simulink model "Failure_generator"  (R2018b)
settings: Solver=VariableStepAuto  StartTime=0.0  StopTime=n_T  RelTol=1e-3
undefined symbols (not defined in the file or in its folder): FM, m, n, WT_n
settings Model: Creator=Jorrit de Jong  LastModifiedBy=Jorrit de Jong

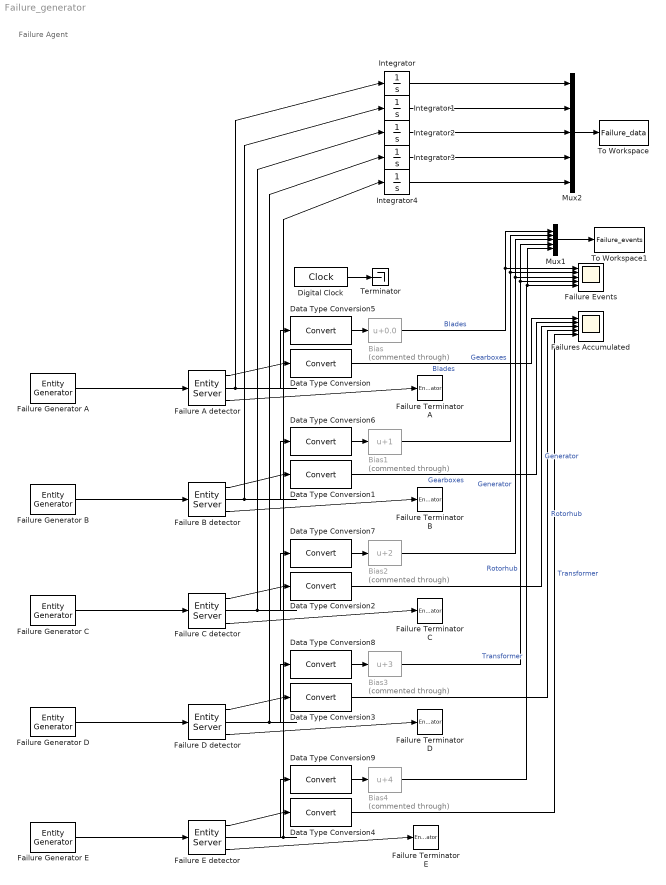
== system Failure_generator ==
  note: Failure Agent
  Bias : Bias  Commented=through  Bias=0.0
  Bias1 : Bias  Commented=through  Bias=1
  Bias2 : Bias  Commented=through  Bias=2
  Bias3 : Bias  Commented=through  Bias=3
  Bias4 : Bias  Commented=through  Bias=4
  Data Type Conversion{,1..9} (10 alike) : DataTypeConversion
  Digital Clock : DigitalClock
  Failure A detector : EntityServer  InputPortMessageModes=m  OutputPortMessageModes=n,n,m  Capacity=1  NumberEntitiesDeparted=on  NumberEntitiesInBlock=on
      settings: OutputPortMap=o0,o1,o9
  Failure B detector : EntityServer  InputPortMessageModes=m  OutputPortMessageModes=n,n,m  Capacity=1  NumberEntitiesDeparted=on  NumberEntitiesInBlock=on
      settings: OutputPortMap=o0,o1,o9
  Failure C detector : EntityServer  InputPortMessageModes=m  OutputPortMessageModes=n,n,m  Capacity=1  NumberEntitiesDeparted=on  NumberEntitiesInBlock=on
      settings: OutputPortMap=o0,o1,o9
  Failure D detector : EntityServer  InputPortMessageModes=m  OutputPortMessageModes=n,n,m  Capacity=1  NumberEntitiesDeparted=on  NumberEntitiesInBlock=on
      settings: OutputPortMap=o0,o1,o9
  Failure E detector : EntityServer  InputPortMessageModes=m  OutputPortMessageModes=n,n,m  Capacity=1  NumberEntitiesDeparted=on  NumberEntitiesInBlock=on
      settings: OutputPortMap=o0,o1,o9
  Failure Events : Scope  NumInputPorts=5
  Failure Generator A : EntityGenerator  OutputPortMessageModes=m  TimeSource=MATLAB action  Period=FM(1,1)*WT_n  IntergenerationTimeAction=|  GenerateEntityAtSimulationStart=off  AttributeName=data  EntityType=Structured  EntityTypeName=Blade
      | persistent rngInit;
      | if isempty(rngInit)
      |     seed = series_seed;
      |     rng(seed);
      |     rngInit = true;
      | end
      | 
      | % Pattern: Gaussian (normal) distribution
      | % m: Mean, d: Standard deviation
      | m = n_T/WT_n/F_blades(1,i); d = n_T/WT_n/F_blades(2,i);
      | dt = abs(m + d * randn);
  Failure Generator B : EntityGenerator  OutputPortMessageModes=m  TimeSource=MATLAB action  IntergenerationTimeAction=|  GenerateEntityAtSimulationStart=off  EntityType=Structured  EntityTypeName=Gearbox
      | persistent rngInit;
      | if isempty(rngInit)
      |     seed = series_seed;
      |     rng(seed);
      |     rngInit = true;
      | end
      | 
      | % Pattern: Gaussian (normal) distribution
      | % m: Mean, d: Standard deviation
      | m = n_T/WT_n/F_gearbox(1,i); d = n_T/WT_n/F_gearbox(2,i);
      | dt = abs(m + d * randn);
  Failure Generator C : EntityGenerator  OutputPortMessageModes=m  TimeSource=MATLAB action  Period=99999999  IntergenerationTimeAction=|  GenerateEntityAtSimulationStart=off  EntityType=Structured  EntityTypeName=Generator
      | persistent rngInit;
      | if isempty(rngInit)
      |     seed = series_seed;
      |     rng(seed);
      |     rngInit = true;
      | end
      | 
      | % Pattern: Gaussian (normal) distribution
      | % m: Mean, d: Standard deviation
      | m = n_T/WT_n/F_generator(1,i); d = n_T/WT_n/F_generator(2,i);
      | dt = abs(m + d * randn);
  Failure Generator D : EntityGenerator  OutputPortMessageModes=m  TimeSource=MATLAB action  Period=9999999  IntergenerationTimeAction=|  GenerateEntityAtSimulationStart=off  EntityType=Structured  EntityTypeName=Rotorhub
      | persistent rngInit;
      | if isempty(rngInit)
      |     seed = series_seed;
      |     rng(seed);
      |     rngInit = true;
      | end
      | 
      | % Pattern: Gaussian (normal) distribution
      | % m: Mean, d: Standard deviation
      | m = n_T/WT_n/F_rotorhub(1,i); d = n_T/WT_n/F_rotorhub(2,i);
      | dt = abs(m + d * randn);
  Failure Generator E : EntityGenerator  OutputPortMessageModes=m  TimeSource=MATLAB action  Period=99999999  IntergenerationTimeAction=|  GenerateEntityAtSimulationStart=off  EntityType=Structured  EntityTypeName=Transformer
      | persistent rngInit;
      | if isempty(rngInit)
      |     seed = series_seed;
      |     rng(seed);
      |     rngInit = true;
      | end
      | 
      | % Pattern: Gaussian (normal) distribution
      | % m: Mean, d: Standard deviation
      | m = n_T/WT_n/F_transformer(1,i); d = n_T/WT_n/F_transformer(2,i);
      | dt = abs(m + d * randn);
  "Failure Terminator A " : EntityTerminator  InputPortMessageModes=m
  Failure Terminator B : EntityTerminator  InputPortMessageModes=m
  Failure Terminator C : EntityTerminator  InputPortMessageModes=m
  Failure Terminator D : EntityTerminator  InputPortMessageModes=m
  Failure Terminator E : EntityTerminator  InputPortMessageModes=m
  Failures Accumulated : Scope  NumInputPorts=5
  Integrator{,1..4} (5 alike) : Integrator
  Mux1 : Mux  Inputs=5
  Mux2 : Mux  Inputs=5
  Terminator : Terminator
  To Workspace : ToWorkspace  VariableName=Failure_data  SaveFormat=Timeseries  SampleTime=1
  To Workspace1 : ToWorkspace  VariableName=Failure_events  SaveFormat=Timeseries  SampleTime=1
  wires:
  Failure A detector/3 -> "Failure Terminator A "/1
  Failure Generator A/1 -> Failure A detector/1
  Failure A detector/1 -> Data Type Conversion/1
  Failure Generator B/1 -> Failure B detector/1
  Failure Generator C/1 -> Failure C detector/1
  Failure Generator D/1 -> Failure D detector/1
  Failure Generator E/1 -> Failure E detector/1
  Failure B detector/3 -> Failure Terminator B/1
  Failure C detector/3 -> Failure Terminator C/1
  Failure D detector/3 -> Failure Terminator D/1
  Failure E detector/3 -> Failure Terminator E/1
  Failure B detector/1 -> Data Type Conversion1/1
  Failure C detector/1 -> Data Type Conversion2/1
  Failure D detector/1 -> Data Type Conversion3/1
  Failure E detector/1 -> Data Type Conversion4/1
  Data Type Conversion/1 -> Failures Accumulated/1  "Blades"
  Data Type Conversion1/1 -> Failures Accumulated/2  "Gearboxes"
  Data Type Conversion2/1 -> Failures Accumulated/3  "Generator"
  Data Type Conversion3/1 -> Failures Accumulated/4  "Rotorhub"
  Data Type Conversion4/1 -> Failures Accumulated/5  "Transformer"
  Failure E detector/2 -> Integrator4/1, Data Type Conversion9/1
  Failure D detector/2 -> Data Type Conversion8/1, Integrator3/1
  Failure C detector/2 -> Data Type Conversion7/1, Integrator2/1
  Failure B detector/2 -> Data Type Conversion6/1, Integrator1/1
  Failure A detector/2 -> Data Type Conversion5/1, Integrator/1
  Data Type Conversion5/1 -> Bias/1
  Data Type Conversion6/1 -> Bias1/1
  Data Type Conversion7/1 -> Bias2/1
  Data Type Conversion8/1 -> Bias3/1
  Data Type Conversion9/1 -> Bias4/1
  Bias/1 -> Mux1/1, Failure Events/1  "Blades"
  Bias1/1 -> Mux1/2, Failure Events/2  "Gearboxes"
  Bias2/1 -> Mux1/3, Failure Events/3  "Generator"
  Bias3/1 -> Mux1/4, Failure Events/4  "Rotorhub"
  Bias4/1 -> Mux1/5, Failure Events/5  "Transformer"
  Mux1/1 -> To Workspace1/1
  Digital Clock/1 -> Terminator/1
  Integrator/1 -> Mux2/1
  Mux2/1 -> To Workspace/1
  Integrator1/1 -> Mux2/2
  Integrator2/1 -> Mux2/3
  Integrator3/1 -> Mux2/4
  Integrator4/1 -> Mux2/5
